simulink library "svm_lib"  (Simulink 8.6)
settings: Solver=VariableStepAuto  StartTime=0.0  StopTime=10.0  RelTol=1e-3
values from neighbouring files (symbols this model uses):
  My_3D = ([eye(6) -eye(6)])    [svm_buildLinearControllers.m]    (also in svm_setup.m = [-eye(6) eye(6)])
  turbulence2loadfactors = blkdiag(T_w2nx, T_w2nz)    [svm_buildLinearControllers.m]
  uavsim = loaded.uavsim    [svm_sandbox.m]
undefined symbols (not defined in the file or in its folder): dt, F, fflib_delay_c2d, Light, mask_p0_NED, mask_v0_NED, MIL, postracking, svm, uavsimblockset_cartesianToAngle
libraries: svm_lib x9, simulink_extras x8, aerolibtransform2 x3, formationFlyingBlockset x2, uavsimBlockset_Cularis_Aerandpropulsion x1, uavsimBlockset_ElectricPropulsion x1, aerolibwind2 x1, aerolibgravity2 x1, uavsimBlockset_VectorNorm x1, uavsimBlockset_UAV3DInterface x1
(part 1 of 3)
settings Model: Creator=j.bolting  LastModifiedBy=j.bolting

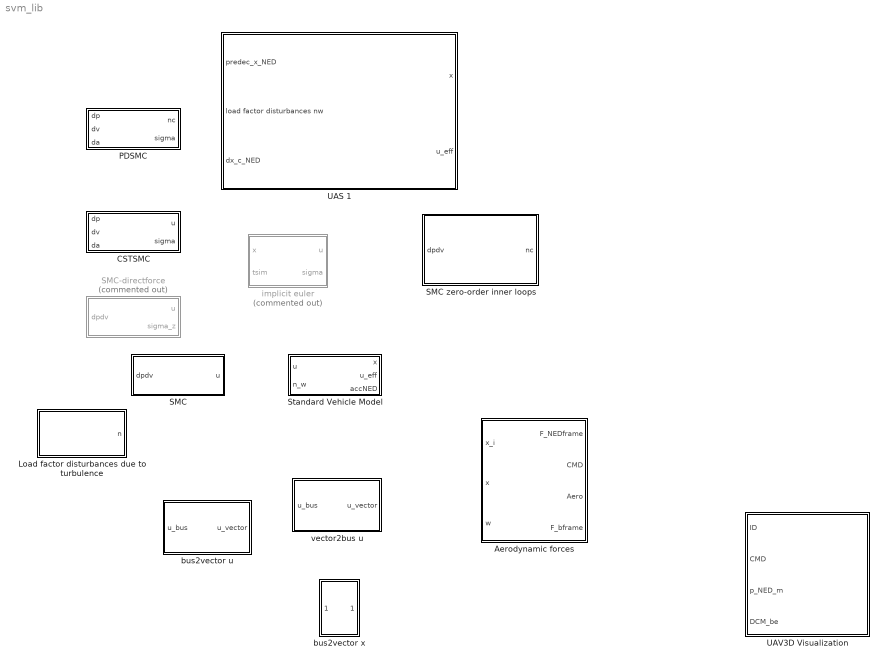
== system svm_lib ==
  Aerodynamic forces : Subsystem
  CSTSMC : Subsystem
  Load factor disturbances due to turbulence : Subsystem
  PDSMC : Subsystem
  SMC : Subsystem
  SMC zero-order inner loops : Subsystem
  SMC-directforce : Subsystem  Commented=on
  Standard Vehicle Model : Subsystem  mask{mask_p0_NED=mask_p0_NED, mask_v0_NED=mask_v0_NED}
      mask prompts: mask_p0_NED "Initial position NED"; mask_v0_NED "Initial velocity NED"
  UAS 1 : Subsystem  mask{mask_vehicleID=1, mask_p0_NED=[0 0 -5], mask_v0_NED=[15 0 0]}
      mask prompts: mask_vehicleID "Vehicle ID"; mask_p0_NED "Initial NED position"; mask_v0_NED "Intial NED speed"
  UAV3D Visualization : Subsystem  AncestorBlock=formationFlyingBlockset/UAV3D Visualization  TreatAsAtomicUnit=on  SystemSampleTime=1/40  mask{mask_visual=2}
      mask prompts: mask_visual "3D model"
      mask TypeOptions mask_visual: 0 | 1 | 2 | 3
  bus2vector u : Subsystem
  bus2vector x : Subsystem
  implicit euler : MATLAB Function  Commented=on  TreatAsAtomicUnit=on  SystemSampleTime=postracking.T
  vector2bus u : Subsystem

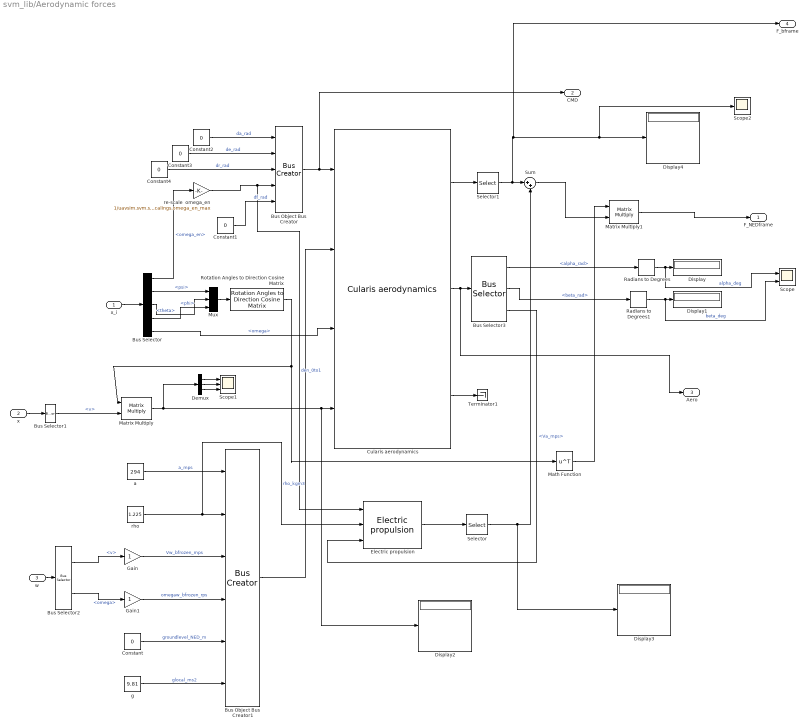
== system svm_lib/Aerodynamic forces ==
  x_i : Inport  OutDataTypeStr=Bus: svm_bus_xi
  x : Inport  Port=2  OutDataTypeStr=Bus: svm_bus_x
  w : Inport  Port=3  OutDataTypeStr=Bus: svm_dwind
  Bus Selector : BusSelector  OutputSignals=omega_en,psi,theta,phi,omega
  Bus Selector1 : BusSelector  OutputSignals=v
  Bus Selector2 : BusSelector  OutputSignals=v,omega
  Bus Selector3 : BusSelector  OutputSignals=alpha_rad,beta_rad,Va_mps
  Bus Object Bus Creator : BusCreator  Inputs=5  OutDataTypeStr=Bus: CMD  mask(BUS OBJECT Bus Creator){busType=Bus: CMD}
      mask prompts: busType "Bus Type"
      mask help:
      | Provides users the cabability to painlessly, instantly customize bus creators of output data type 'Bus:' by selecting the bus object type from a drop down menu dynamically populated by bus objects in the workspace.
      |
      | After pressing the "Apply Selection" button signal lines into the creator are populated and named with the elements in the chosen bus saving the user from having to recall and fill out signal line names.
      |
      | NOTE that when copying a Bus Object Bus Creator from your locked Library the link to the Library is automatically broken. This saves the user from having to Unlock Links To Library (From the Library menu.), Disable Link and finally Break Link (Both from the Model menu.) for every placed instance of the block.
      settings: AttributesFormatString=%<OutDataTypeStr>  CopyFcn=set_param(gcb, 'LinkStatus', 'none')
      mask TypeOptions busType: Bus: AHRS | Bus: Acceleration | Bus: Aero | Bus: Airdata | Bus: Airframe | Bus: Attitude | Bus: CMD | Bus: CMD_quadrotor | Bus: ControlInfoBus | Bus: Enginedata | Bus: Environment | Bus: FlightGearData | Bus: GCSUpstream | Bus: GNSSL1 | Bus: GNSSRTK | Bus: GPS | Bus: IMU | Bus: Kinematics | Bus: LandinggearInput | Bus: MotionTracker | Bus: Position | Bus: Radiodistance | Bus: RotationalAcceleration | Bus: RotationalVelocity | Bus: SensorBus | Bus: StateBus | Bus: Velocity | Bus: WindAngles | Bus: iUAScom | Bus: slBus1 | Bus: svm_bus_u_scaled | Bus: svm_bus_x | Bus: svm_bus_xi | Bus: svm_dwind
      mask Callback busType:
      | % Using variable names terminated with "_BOBC" to lessen the chances of
      | % collisions with existing workspace variables.
      | 
      | % Get the current block handle and mask handle.
      | handleCreator_BOBC = gcbh;
      | maskObj_BOBC       = Simulink.Mask.get(gcb);
      | 
      | % Get a list of variables in the workspace in order to search for the '1x1
      | % Bus' types.
      | wsVars_BOBC = whos;
      | 
      | % Reset the 'TypeOptions' bus list in case some '1x1 Bus' types have been
      | % deleted from or added to the workspace.
      | maskObj_BOBC.Parameters.TypeOptions = {'<empty>'};
      | 
      | % Reset the bus count.
      | busCount_BOBC = 0;
      | 
      | for index_BOBC = 1:length(wsVars_BOBC)
      | 
      |    % If the variable is a bus object...
      |    if strcmp(wsVars_BOBC(index_BOBC).class, 'Simulink.Bus')
      | 
      |       busCount_BOBC = busCount_BOBC + 1;
      | 
      |       % ... add it to the TypeOptions of the mask.
      |       maskObj_BOBC.Parameters.TypeOptions(busCount_BOBC) = ...
      |                                                            ...
      |                                  {['Bus: ', wsVars_BOBC(index_BOBC).name]};
      |    end
      | end
      | 
      | if busCount_BOBC == 0
      | 
      |    % If there are NO bus objects in the workspace then provide a warning
      |    % popup...
      |    warndlg('There are currently no bus objects in the workspace - you have no use for this block. Use a normal Bus Creator instead.')
      | 
      |    % ... and do nothing.
      | elseif ~strcmp(get_param(handleCreator_BOBC, 'OutDataTypeStr'), 'Inherit: auto')
      | 
      |    % If the currently selected bus data type ('OutDataTypeStr') is not
      |    % 'Inherit: auto' (i.e., if we are reopening the mask.) then get the
      |    % current 'OutDataTypeStr' and 'maskVal.' ('maskVal' is the selected
      |    % 'TypeOptions' list member.)
      |    outDatStr_BOBC = get_param(handleCreator_BOBC, 'OutDataTypeStr');
      |    maskVal_BOBC   = get_param(handleCreator_BOBC, 'MaskValues');
      | 
      |    if ~strcmp(outDatStr_BOBC, maskVal_BOBC{1})
      | 
      |       % Upon re-opening the mask if the default 'TypeOptions' list member
      |       % (The first one.) contained in 'maskVal' does not match the
      |       % currently selected bus data type ('OutDataTypeStr') then set the
      |       % 'TypeOptions' list member to the selected bus data type. (Cuts down
      |       % on confusion to have the displayed list member match the selected
      |       % bus data type rather than the first entry.)
      |       set_param(handleCreator_BOBC, 'MaskValues', {outDatStr_BOBC});
      |    end
      | end
      | 
      | % Clean up the workspace.
      | clear  handleCreator_BOBC  maskObj_BOBC     wsVars_BOBC ...
      |             busCount_BOBC    index_BOBC  outDatStr_BOBC ...
      |              maskVal_BOBC
      mask DialogControl applyMOCBSelection Prompt: Apply Selection
      mask DialogControl applyMOCBSelection Callback:
      | % Using variable names terminated with "_BOBC" to lessen the chances of
      | % collisions with existing workspace variables.
      | 
      | % Get the current block, current block handle and mask handle.
      | currentBlock_BOBC  = gcb;
      | handleCreator_BOBC = gcbh;
      | 
      | % Get the desired bus type...
      | desiredBusType_BOBC = get_param(handleCreator_BOBC, 'busType');
      | 
      | % ... and set the 'OutDataTypeStr' to it.
      | set_param(handleCreator_BOBC, 'OutDataTypeStr', desiredBusType_BOBC);
      | 
      | %% First delete any existing lines on the port.
      | % Get the line handles.
      | lh_BOBC = get_param(handleCreator_BOBC, 'LineHandles');
      | 
      | % If any lines exist (Non- -1 line handles.), delete them and start over.
      | if max(lh_BOBC.Inport > 0)
      | 
      |    for index_BOBC = 1:length(lh_BOBC.Inport)
      | 
      |       if lh_BOBC.Inport(index_BOBC) > 0
      | 
      |          delete_line(lh_BOBC.Inport(index_BOBC))
      |       end
      |    end
      | end
      | 
      | %% Then work on adding new lines.
      | 
      | % Get the block path for 'add_line' function.
      | blockPath_BOBC = get_param(handleCreator_BOBC, 'Parent');
      | 
      | % Get the newly selected bus type ('OutDataTypeStr')...
      | mocbBusType_BOBC = get_param(currentBlock_BOBC, 'OutDataTypeStr');
      | 
      | % ... and parse off "Bus: " so the string of the desired bus contained in
      | % 'OutDataTypeStr' matches the raw workspace bus names.
      | mocbBusType_BOBC = mocbBusType_BOBC(6:end);
      | 
      | % Then evaluate the string containing the workspace bus name which will
      | % load the desired bus parameters.
      | busParams_BOBC = eval(mocbBusType_BOBC);
      | 
      | % From the parameters grab the number of lines to add.
      | numLines_BOBC = length(busParams_BOBC.Elements);
      | 
      | % Set the number of inputs of the masked bus creator to the number of lines
      | % to add.
      | set_param(handleCreator_BOBC, 'Inputs', num2str(numLines_BOBC));
      | 
      | % Get (Inputs.) port handles so we can grab the positions of them.
      | ph_BOBC = get_param(handleCreator_BOBC, 'PortHandles');
      | 
      | for index_BOBC = 1:numLines_BOBC
      | 
      |    % Get the position of input port number 'index_BOBC'.
      |    portPos_BOBC = get_param(ph_BOBC.Inport(index_BOBC), 'Position');
      | 
      |    % Add a line from 50 pixels left of the port position to the port
      |    % position. (This must be done because it's the lines that get named,
      |    % not the port positions.)
      |    portLine_BOBC = add_line(blockPath_BOBC, [portPos_BOBC - [50 0]; portPos_BOBC]);
      | 
      |    % Rename the new line to the bus 'index_BOBC-st/nd/rd/th' element name.
      |    set_param(portLine_BOBC, 'Name', busParams_BOBC.Elements(index_BOBC).Name)
      | end
      | 
      | %% Cleanup the workspace.
      | clear    currentBlock_BOBC  handleCreator_BOBC      index_BOBC ...
      |        desiredBusType_BOBC             lh_BOBC  blockPath_BOBC ...
      |           mocbBusType_BOBC      busParams_BOBC   numLines_BOBC ...
      |                    ph_BOBC        portPos_BOBC   portLine_BOBC
  Bus Object Bus Creator1 : BusCreator  Inputs=6  OutDataTypeStr=Bus: Environment  mask(BUS OBJECT Bus Creator){busType=Bus: Environment}
      mask prompts: busType "Bus Type"
      mask help:
      | Provides users the cabability to painlessly, instantly customize bus creators of output data type 'Bus:' by selecting the bus object type from a drop down menu dynamically populated by bus objects in the workspace.
      |
      | After pressing the "Apply Selection" button signal lines into the creator are populated and named with the elements in the chosen bus saving the user from having to recall and fill out signal line names.
      |
      | NOTE that when copying a Bus Object Bus Creator from your locked Library the link to the Library is automatically broken. This saves the user from having to Unlock Links To Library (From the Library menu.), Disable Link and finally Break Link (Both from the Model menu.) for every placed instance of the block.
      settings: AttributesFormatString=%<OutDataTypeStr>  CopyFcn=set_param(gcb, 'LinkStatus', 'none')
      mask TypeOptions busType: Bus: AHRS | Bus: Acceleration | Bus: Aero | Bus: Airdata | Bus: Airframe | Bus: Attitude | Bus: CMD | Bus: CMD_quadrotor | Bus: ControlInfoBus | Bus: Enginedata | Bus: Environment | Bus: FlightGearData | Bus: GCSUpstream | Bus: GNSSL1 | Bus: GNSSRTK | Bus: GPS | Bus: IMU | Bus: Kinematics | Bus: LandinggearInput | Bus: MotionTracker | Bus: Position | Bus: Radiodistance | Bus: RotationalAcceleration | Bus: RotationalVelocity | Bus: SensorBus | Bus: StateBus | Bus: Velocity | Bus: WindAngles | Bus: iUAScom | Bus: slBus1 | Bus: svm_bus_u_scaled | Bus: svm_bus_x | Bus: svm_bus_xi | Bus: svm_dwind
      mask Callback busType:
      | % Using variable names terminated with "_BOBC" to lessen the chances of
      | % collisions with existing workspace variables.
      | 
      | % Get the current block handle and mask handle.
      | handleCreator_BOBC = gcbh;
      | maskObj_BOBC       = Simulink.Mask.get(gcb);
      | 
      | % Get a list of variables in the workspace in order to search for the '1x1
      | % Bus' types.
      | wsVars_BOBC = whos;
      | 
      | % Reset the 'TypeOptions' bus list in case some '1x1 Bus' types have been
      | % deleted from or added to the workspace.
      | maskObj_BOBC.Parameters.TypeOptions = {'<empty>'};
      | 
      | % Reset the bus count.
      | busCount_BOBC = 0;
      | 
      | for index_BOBC = 1:length(wsVars_BOBC)
      | 
      |    % If the variable is a bus object...
      |    if strcmp(wsVars_BOBC(index_BOBC).class, 'Simulink.Bus')
      | 
      |       busCount_BOBC = busCount_BOBC + 1;
      | 
      |       % ... add it to the TypeOptions of the mask.
      |       maskObj_BOBC.Parameters.TypeOptions(busCount_BOBC) = ...
      |                                                            ...
      |                                  {['Bus: ', wsVars_BOBC(index_BOBC).name]};
      |    end
      | end
      | 
      | if busCount_BOBC == 0
      | 
      |    % If there are NO bus objects in the workspace then provide a warning
      |    % popup...
      |    warndlg('There are currently no bus objects in the workspace - you have no use for this block. Use a normal Bus Creator instead.')
      | 
      |    % ... and do nothing.
      | elseif ~strcmp(get_param(handleCreator_BOBC, 'OutDataTypeStr'), 'Inherit: auto')
      | 
      |    % If the currently selected bus data type ('OutDataTypeStr') is not
      |    % 'Inherit: auto' (i.e., if we are reopening the mask.) then get the
      |    % current 'OutDataTypeStr' and 'maskVal.' ('maskVal' is the selected
      |    % 'TypeOptions' list member.)
      |    outDatStr_BOBC = get_param(handleCreator_BOBC, 'OutDataTypeStr');
      |    maskVal_BOBC   = get_param(handleCreator_BOBC, 'MaskValues');
      | 
      |    if ~strcmp(outDatStr_BOBC, maskVal_BOBC{1})
      | 
      |       % Upon re-opening the mask if the default 'TypeOptions' list member
      |       % (The first one.) contained in 'maskVal' does not match the
      |       % currently selected bus data type ('OutDataTypeStr') then set the
      |       % 'TypeOptions' list member to the selected bus data type. (Cuts down
      |       % on confusion to have the displayed list member match the selected
      |       % bus data type rather than the first entry.)
      |       set_param(handleCreator_BOBC, 'MaskValues', {outDatStr_BOBC});
      |    end
      | end
      | 
      | % Clean up the workspace.
      | clear  handleCreator_BOBC  maskObj_BOBC     wsVars_BOBC ...
      |             busCount_BOBC    index_BOBC  outDatStr_BOBC ...
      |              maskVal_BOBC
      mask DialogControl applyMOCBSelection Prompt: Apply Selection
      mask DialogControl applyMOCBSelection Callback:
      | % Using variable names terminated with "_BOBC" to lessen the chances of
      | % collisions with existing workspace variables.
      | 
      | % Get the current block, current block handle and mask handle.
      | currentBlock_BOBC  = gcb;
      | handleCreator_BOBC = gcbh;
      | 
      | % Get the desired bus type...
      | desiredBusType_BOBC = get_param(handleCreator_BOBC, 'busType');
      | 
      | % ... and set the 'OutDataTypeStr' to it.
      | set_param(handleCreator_BOBC, 'OutDataTypeStr', desiredBusType_BOBC);
      | 
      | %% First delete any existing lines on the port.
      | % Get the line handles.
      | lh_BOBC = get_param(handleCreator_BOBC, 'LineHandles');
      | 
      | % If any lines exist (Non- -1 line handles.), delete them and start over.
      | if max(lh_BOBC.Inport > 0)
      | 
      |    for index_BOBC = 1:length(lh_BOBC.Inport)
      | 
      |       if lh_BOBC.Inport(index_BOBC) > 0
      | 
      |          delete_line(lh_BOBC.Inport(index_BOBC))
      |       end
      |    end
      | end
      | 
      | %% Then work on adding new lines.
      | 
      | % Get the block path for 'add_line' function.
      | blockPath_BOBC = get_param(handleCreator_BOBC, 'Parent');
      | 
      | % Get the newly selected bus type ('OutDataTypeStr')...
      | mocbBusType_BOBC = get_param(currentBlock_BOBC, 'OutDataTypeStr');
      | 
      | % ... and parse off "Bus: " so the string of the desired bus contained in
      | % 'OutDataTypeStr' matches the raw workspace bus names.
      | mocbBusType_BOBC = mocbBusType_BOBC(6:end);
      | 
      | % Then evaluate the string containing the workspace bus name which will
      | % load the desired bus parameters.
      | busParams_BOBC = eval(mocbBusType_BOBC);
      | 
      | % From the parameters grab the number of lines to add.
      | numLines_BOBC = length(busParams_BOBC.Elements);
      | 
      | % Set the number of inputs of the masked bus creator to the number of lines
      | % to add.
      | set_param(handleCreator_BOBC, 'Inputs', num2str(numLines_BOBC));
      | 
      | % Get (Inputs.) port handles so we can grab the positions of them.
      | ph_BOBC = get_param(handleCreator_BOBC, 'PortHandles');
      | 
      | for index_BOBC = 1:numLines_BOBC
      | 
      |    % Get the position of input port number 'index_BOBC'.
      |    portPos_BOBC = get_param(ph_BOBC.Inport(index_BOBC), 'Position');
      | 
      |    % Add a line from 50 pixels left of the port position to the port
      |    % position. (This must be done because it's the lines that get named,
      |    % not the port positions.)
      |    portLine_BOBC = add_line(blockPath_BOBC, [portPos_BOBC - [50 0]; portPos_BOBC]);
      | 
      |    % Rename the new line to the bus 'index_BOBC-st/nd/rd/th' element name.
      |    set_param(portLine_BOBC, 'Name', busParams_BOBC.Elements(index_BOBC).Name)
      | end
      | 
      | %% Cleanup the workspace.
      | clear    currentBlock_BOBC  handleCreator_BOBC      index_BOBC ...
      |        desiredBusType_BOBC             lh_BOBC  blockPath_BOBC ...
      |           mocbBusType_BOBC      busParams_BOBC   numLines_BOBC ...
      |                    ph_BOBC        portPos_BOBC   portLine_BOBC
  Constant{,1..4} (5 alike) : Constant  Value=0
  Cularis aerodynamics : uavsimBlockset_Cularis_Aerandpropulsion/Cularis aerodynamics  SystemSampleTime=-1
  Demux : Demux  Outputs=3
  Display{,1..4} (5 alike) : Display
  Electric propulsion : uavsimBlockset_ElectricPropulsion/Electric propulsion  mask_C_prop=uavsim.zagi.engine.C_prop  mask_S_prop=uavsim.zagi.engine.S_prop  mask_k_motor=uavsim.zagi.engine.k_motor
  Gain : Gain
  Gain1 : Gain
  Math Function : Math  Operator=transpose  SaturateOnIntegerOverflow=on
  Matrix Multiply : Product  Multiplication=Matrix(*)
  Matrix Multiply1 : Product  Multiplication=Matrix(*)
  Mux : Mux  Inputs=3
  Radians to Degrees : simulink_extras/Transformations/Radians to Degrees
  Radians to Degrees1 : simulink_extras/Transformations/Radians to Degrees
  Rotation Angles to Direction Cosine Matrix : aerolibtransform2/Rotation Angles to Direction Cosine Matrix  rotationOrder=ZYX
  Scope : Scope  NumInputPorts=2
  Scope1 : Scope  NumInputPorts=3
  Scope2 : Scope
  Selector : Selector  InputPortWidth=6  IndexOptions=Index vector (dialog)  Indices=1:3  OutputSizes=1
  Selector1 : Selector  InputPortWidth=6  IndexOptions=Index vector (dialog)  Indices=1:3  OutputSizes=1
  Sum : Sum  Inputs=|++
  Terminator1 : Terminator
  a : Constant  Value=294
  g : Constant  Value=9.81
  re-scale  omega_en : Gain  Gain=1/uavsim.svm.scalings.omega_en_max
  "rho " : Constant  Value=1.225
  F_NEDframe : Outport
  CMD : Outport  Port=2  OutDataTypeStr=Bus: CMD
  Aero : Outport  Port=3  OutDataTypeStr=Bus: Aero
  F_bframe : Outport  Port=4
  wires:
  Selector1/1 -> Sum/1, Display4/1, Scope2/1, F_bframe/1
  Demux/3 -> Scope1/3
  Demux/1 -> Scope1/1
  Demux/2 -> Scope1/2
  Radians to Degrees1/1 -> Display1/1, Scope/2  "beta_deg"
  Radians to Degrees/1 -> Display/1, Scope/1  "alpha_deg"
  Bus Selector3/2 -> Radians to Degrees1/1  "<beta_rad>"
  Bus Selector3/1 -> Radians to Degrees/1  "<alpha_rad>"
  Bus Selector3/3 -> Electric propulsion/3  "<Va_mps>"
  Bus Selector2/1 -> Gain/1  "<v>"
  Bus Selector2/2 -> Gain1/1  "<omega>"
  Bus Object Bus Creator/1 -> CMD/1, Cularis aerodynamics/1
  Constant2/1 -> Bus Object Bus Creator/1  "da_rad"
  Constant3/1 -> Bus Object Bus Creator/2  "de_rad"
  Constant4/1 -> Bus Object Bus Creator/3  "dr_rad"
  re-scale  omega_en/1 -> Electric propulsion/1, Bus Object Bus Creator/4  "den_0to1"
  Constant1/1 -> Bus Object Bus Creator/5  "df_rad"
  x_i/1 -> Bus Selector/1
  Bus Selector/1 -> re-scale  omega_en/1  "<omega_en>"
  Bus Selector/2 -> Mux/1  "<psi>"
  Cularis aerodynamics/2 -> Aero/1, Bus Selector3/1
  Cularis aerodynamics/3 -> Terminator1/1
  Electric propulsion/1 -> Selector/1
  Matrix Multiply1/1 -> F_NEDframe/1
  Selector/1 -> Sum/2, Display3/1
  Cularis aerodynamics/1 -> Selector1/1
  Bus Selector/5 -> Cularis aerodynamics/3  "<omega>"
  Bus Selector/4 -> Mux/3  "<phi>"
  Bus Selector/3 -> Mux/2  "<theta>"
  Mux/1 -> Rotation Angles to Direction Cosine Matrix/1
  a/1 -> Bus Object Bus Creator1/1  "a_mps"
  "rho "/1 -> Electric propulsion/2, Bus Object Bus Creator1/2  "rho_kgm3"
  Gain/1 -> Bus Object Bus Creator1/3  "Vw_bfrozen_mps"
  Gain1/1 -> Bus Object Bus Creator1/4  "omegaw_bfrozen_rps"
  Constant/1 -> Bus Object Bus Creator1/5  "groundlevel_NED_m"
  g/1 -> Bus Object Bus Creator1/6  "glocal_ms2"
  w/1 -> Bus Selector2/1
  Bus Object Bus Creator1/1 -> Cularis aerodynamics/2
  x/1 -> Bus Selector1/1
  Bus Selector1/1 -> Matrix Multiply/2  "<v>"
  Matrix Multiply/1 -> Cularis aerodynamics/4, Display2/1, Demux/1
  Rotation Angles to Direction Cosine Matrix/1 -> Math Function/1, Matrix Multiply/1
  Math Function/1 -> Matrix Multiply1/1
  Sum/1 -> Matrix Multiply1/2

== system svm_lib/CSTSMC ==
  dp : Inport
  dv : Inport  Port=2
  da : Inport  Port=3
  Integrator : Integrator
  MATLAB Function : MATLAB Function  TreatAsAtomicUnit=on
  Scope : Scope
  Sum : Sum  Inputs=|++
  Zero-Order Hold : ZeroOrderHold  SampleTime=postracking.T
  u : Outport
  sigma : Outport  Port=2
  wires:
  da/1 -> MATLAB Function/3(da)
  Sum/1 -> Zero-Order Hold/1, MATLAB Function/4(u)
  Zero-Order Hold/1 -> u/1
  dv/1 -> MATLAB Function/2(dv)
  MATLAB Function/3(sigma) -> sigma/1
  Integrator/1 -> Sum/2
  MATLAB Function/1(u1) -> Sum/1, Scope/1
  MATLAB Function/2(w) -> Integrator/1
  dp/1 -> MATLAB Function/1(dp)

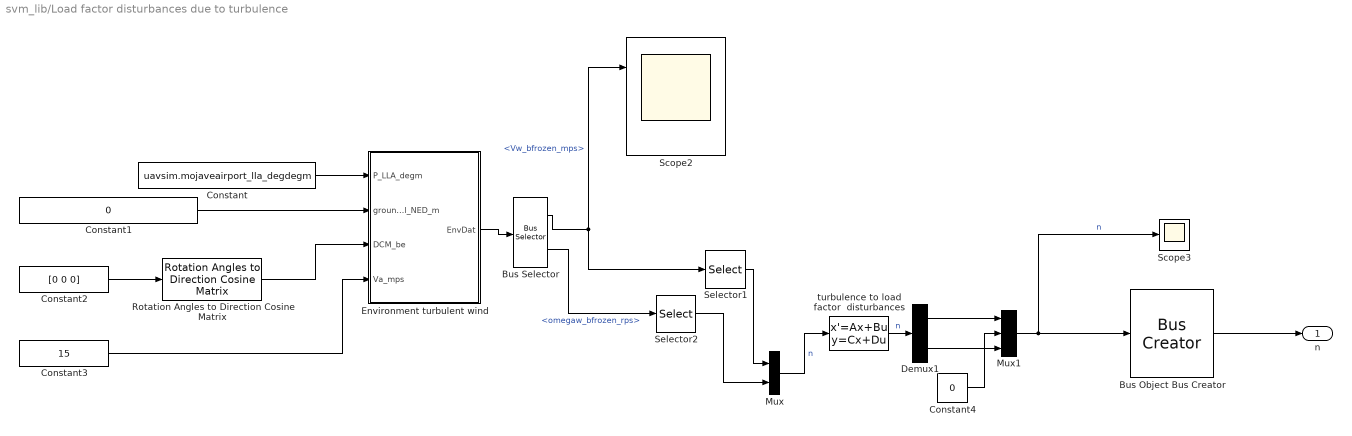
== system svm_lib/Load factor disturbances due to turbulence ==
  Bus Selector : BusSelector  OutputSignals=Vw_bfrozen_mps,omegaw_bfrozen_rps
  Bus Object Bus Creator : BusCreator  Inputs=1  OutDataTypeStr=Bus: svm_bus_u_scaled  mask(BUS OBJECT Bus Creator){busType=Bus: svm_bus_u_scaled}
      mask prompts: busType "Bus Type"
      mask help:
      | Provides users the cabability to painlessly, instantly customize bus creators of output data type 'Bus:' by selecting the bus object type from a drop down menu dynamically populated by bus objects in the workspace.
      |
      | After pressing the "Apply Selection" button signal lines into the creator are populated and named with the elements in the chosen bus saving the user from having to recall and fill out signal line names.
      |
      | NOTE that when copying a Bus Object Bus Creator from your locked Library the link to the Library is automatically broken. This saves the user from having to Unlock Links To Library (From the Library menu.), Disable Link and finally Break Link (Both from the Model menu.) for every placed instance of the block.
      settings: AttributesFormatString=%<OutDataTypeStr>  CopyFcn=set_param(gcb, 'LinkStatus', 'none')
      mask TypeOptions busType: Bus: AHRS | Bus: Acceleration | Bus: Aero | Bus: Airdata | Bus: Airframe | Bus: Attitude | Bus: CMD | Bus: CMD_quadrotor | Bus: ControlInfoBus | Bus: Enginedata | Bus: Environment | Bus: FlightGearData | Bus: GCSUpstream | Bus: GNSSL1 | Bus: GNSSRTK | Bus: GPS | Bus: IMU | Bus: Kinematics | Bus: LandinggearInput | Bus: MotionTracker | Bus: Position | Bus: Radiodistance | Bus: RotationalAcceleration | Bus: RotationalVelocity | Bus: SensorBus | Bus: StateBus | Bus: Velocity | Bus: WindAngles | Bus: iUAScom | Bus: svm_bus_d_exo | Bus: svm_bus_u_scaled | Bus: svm_bus_x | Bus: svm_bus_xi
      mask Callback busType:
      | % Using variable names terminated with "_BOBC" to lessen the chances of
      | % collisions with existing workspace variables.
      | 
      | % Get the current block handle and mask handle.
      | handleCreator_BOBC = gcbh;
      | maskObj_BOBC       = Simulink.Mask.get(gcb);
      | 
      | % Get a list of variables in the workspace in order to search for the '1x1
      | % Bus' types.
      | wsVars_BOBC = whos;
      | 
      | % Reset the 'TypeOptions' bus list in case some '1x1 Bus' types have been
      | % deleted from or added to the workspace.
      | maskObj_BOBC.Parameters.TypeOptions = {'<empty>'};
      | 
      | % Reset the bus count.
      | busCount_BOBC = 0;
      | 
      | for index_BOBC = 1:length(wsVars_BOBC)
      | 
      |    % If the variable is a bus object...
      |    if strcmp(wsVars_BOBC(index_BOBC).class, 'Simulink.Bus')
      | 
      |       busCount_BOBC = busCount_BOBC + 1;
      | 
      |       % ... add it to the TypeOptions of the mask.
      |       maskObj_BOBC.Parameters.TypeOptions(busCount_BOBC) = ...
      |                                                            ...
      |                                  {['Bus: ', wsVars_BOBC(index_BOBC).name]};
      |    end
      | end
      | 
      | if busCount_BOBC == 0
      | 
      |    % If there are NO bus objects in the workspace then provide a warning
      |    % popup...
      |    warndlg('There are currently no bus objects in the workspace - you have no use for this block. Use a normal Bus Creator instead.')
      | 
      |    % ... and do nothing.
      | elseif ~strcmp(get_param(handleCreator_BOBC, 'OutDataTypeStr'), 'Inherit: auto')
      | 
      |    % If the currently selected bus data type ('OutDataTypeStr') is not
      |    % 'Inherit: auto' (i.e., if we are reopening the mask.) then get the
      |    % current 'OutDataTypeStr' and 'maskVal.' ('maskVal' is the selected
      |    % 'TypeOptions' list member.)
      |    outDatStr_BOBC = get_param(handleCreator_BOBC, 'OutDataTypeStr');
      |    maskVal_BOBC   = get_param(handleCreator_BOBC, 'MaskValues');
      | 
      |    if ~strcmp(outDatStr_BOBC, maskVal_BOBC{1})
      | 
      |       % Upon re-opening the mask if the default 'TypeOptions' list member
      |       % (The first one.) contained in 'maskVal' does not match the
      |       % currently selected bus data type ('OutDataTypeStr') then set the
      |       % 'TypeOptions' list member to the selected bus data type. (Cuts down
      |       % on confusion to have the displayed list member match the selected
      |       % bus data type rather than the first entry.)
      |       set_param(handleCreator_BOBC, 'MaskValues', {outDatStr_BOBC});
      |    end
      | end
      | 
      | % Clean up the workspace.
      | clear  handleCreator_BOBC  maskObj_BOBC     wsVars_BOBC ...
      |             busCount_BOBC    index_BOBC  outDatStr_BOBC ...
      |              maskVal_BOBC
      mask DialogControl applyMOCBSelection Prompt: Apply Selection
      mask DialogControl applyMOCBSelection Callback:
      | % Using variable names terminated with "_BOBC" to lessen the chances of
      | % collisions with existing workspace variables.
      | 
      | % Get the current block, current block handle and mask handle.
      | currentBlock_BOBC  = gcb;
      | handleCreator_BOBC = gcbh;
      | 
      | % Get the desired bus type...
      | desiredBusType_BOBC = get_param(handleCreator_BOBC, 'busType');
      | 
      | % ... and set the 'OutDataTypeStr' to it.
      | set_param(handleCreator_BOBC, 'OutDataTypeStr', desiredBusType_BOBC);
      | 
      | %% First delete any existing lines on the port.
      | % Get the line handles.
      | lh_BOBC = get_param(handleCreator_BOBC, 'LineHandles');
      | 
      | % If any lines exist (Non- -1 line handles.), delete them and start over.
      | if max(lh_BOBC.Inport > 0)
      | 
      |    for index_BOBC = 1:length(lh_BOBC.Inport)
      | 
      |       if lh_BOBC.Inport(index_BOBC) > 0
      | 
      |          delete_line(lh_BOBC.Inport(index_BOBC))
      |       end
      |    end
      | end
      | 
      | %% Then work on adding new lines.
      | 
      | % Get the block path for 'add_line' function.
      | blockPath_BOBC = get_param(handleCreator_BOBC, 'Parent');
      | 
      | % Get the newly selected bus type ('OutDataTypeStr')...
      | mocbBusType_BOBC = get_param(currentBlock_BOBC, 'OutDataTypeStr');
      | 
      | % ... and parse off "Bus: " so the string of the desired bus contained in
      | % 'OutDataTypeStr' matches the raw workspace bus names.
      | mocbBusType_BOBC = mocbBusType_BOBC(6:end);
      | 
      | % Then evaluate the string containing the workspace bus name which will
      | % load the desired bus parameters.
      | busParams_BOBC = eval(mocbBusType_BOBC);
      | 
      | % From the parameters grab the number of lines to add.
      | numLines_BOBC = length(busParams_BOBC.Elements);
      | 
      | % Set the number of inputs of the masked bus creator to the number of lines
      | % to add.
      | set_param(handleCreator_BOBC, 'Inputs', num2str(numLines_BOBC));
      | 
      | % Get (Inputs.) port handles so we can grab the positions of them.
      | ph_BOBC = get_param(handleCreator_BOBC, 'PortHandles');
      | 
      | for index_BOBC = 1:numLines_BOBC
      | 
      |    % Get the position of input port number 'index_BOBC'.
      |    portPos_BOBC = get_param(ph_BOBC.Inport(index_BOBC), 'Position');
      | 
      |    % Add a line from 50 pixels left of the port position to the port
      |    % position. (This must be done because it's the lines that get named,
      |    % not the port positions.)
      |    portLine_BOBC = add_line(blockPath_BOBC, [portPos_BOBC - [50 0]; portPos_BOBC]);
      | 
      |    % Rename the new line to the bus 'index_BOBC-st/nd/rd/th' element name.
      |    set_param(portLine_BOBC, 'Name', busParams_BOBC.Elements(index_BOBC).Name)
      | end
      | 
      | %% Cleanup the workspace.
      | clear    currentBlock_BOBC  handleCreator_BOBC      index_BOBC ...
      |        desiredBusType_BOBC             lh_BOBC  blockPath_BOBC ...
      |           mocbBusType_BOBC      busParams_BOBC   numLines_BOBC ...
      |                    ph_BOBC        portPos_BOBC   portLine_BOBC
  Constant : Constant  Value=uavsim.mojaveairport_lla_degdegm
  Constant1 : Constant  Value=0
  Constant2 : Constant  Value=[0 0 0]
  Constant3 : Constant  Value=15
  Constant4 : Constant  Value=0
  Demux1 : Demux  Outputs=2
  Environment turbulent wind : Subsystem  AncestorBlock=uavsimBlockset_Environment_turbulentWind/Environment turbulent wind  mask{mask_constantwind_NED_mps=svm.ambientWind, mask_wingspan=uavsim.cularis.b, mask_windON=svm.ambientWindOn, mask_turbulenceON=svm.turbulenceOn}
      mask prompts: mask_constantwind_NED_mps "Ambient, i.e. constant wind vector [m/s], NED frame"; mask_wingspan "Aircraft wingspan"; mask_windON "Ambient wind ON?"; mask_turbulenceON "Turbulence ON?"
  Mux : Mux  Inputs=2
  Mux1 : Mux  Inputs=3
  Rotation Angles to Direction Cosine Matrix : aerolibtransform2/Rotation Angles to Direction Cosine Matrix  rotationOrder=ZYX
  Scope2 : Scope  NumInputPorts=2
  Scope3 : Scope
  Selector1 : Selector  InputPortWidth=3  IndexOptions=Index vector (dialog)  Indices=[1 3]  OutputSizes=1
  Selector2 : Selector  InputPortWidth=3  IndexOptions=Index vector (dialog)  Indices=2  OutputSizes=1
  turbulence to load factor  disturbances : StateSpace  A=turbulence2loadfactors.a  B=turbulence2loadfactors.b  C=turbulence2loadfactors.c  D=turbulence2loadfactors.d  X0=0
  n : Outport
  wires:
  Selector1/1 -> Mux/1
  Mux/1 -> turbulence to load factor  disturbances/1  "n"
  Bus Object Bus Creator/1 -> n/1
  Constant3/1 -> Environment turbulent wind/4(Va_mps)
  Environment turbulent wind/1(EnvDat) -> Bus Selector/1
  Bus Selector/2 -> Selector2/1  "<omegaw_bfrozen_rps>"
  Rotation Angles to Direction Cosine Matrix/1 -> Environment turbulent wind/3(DCM_be)
  Bus Selector/1 -> Selector1/1, Scope2/1  "<Vw_bfrozen_mps>"
  Constant/1 -> Environment turbulent wind/1(P_LLA_degm)
  Demux1/1 -> Mux1/1
  Constant1/1 -> Environment turbulent wind/2(groundlevel_NED_m)
  turbulence to load factor  disturbances/1 -> Demux1/1  "n"
  Constant2/1 -> Rotation Angles to Direction Cosine Matrix/1
  Selector2/1 -> Mux/2
  Mux1/1 -> Scope3/1, Bus Object Bus Creator/1  "n"
  Demux1/2 -> Mux1/3
  Constant4/1 -> Mux1/2

== system svm_lib/PDSMC ==
  dp : Inport
  dv : Inport  Port=2
  da : Inport  Port=3
  Digital Clock : DigitalClock  SampleTime=-1
  MATLAB Function : MATLAB Function  TreatAsAtomicUnit=on  SystemSampleTime=postracking.T
  Scope : Scope
  Scope1 : Scope
  nc : Outport
  sigma : Outport  Port=2
  wires:
  Digital Clock/1 -> MATLAB Function/4(tsim)
  MATLAB Function/3(dbport) -> Scope1/1
  dp/1 -> MATLAB Function/1(dp)
  MATLAB Function/2(sigma) -> sigma/1
  dv/1 -> MATLAB Function/2(dv)
  MATLAB Function/1(nc) -> Scope/1, nc/1
  da/1 -> MATLAB Function/3(da)

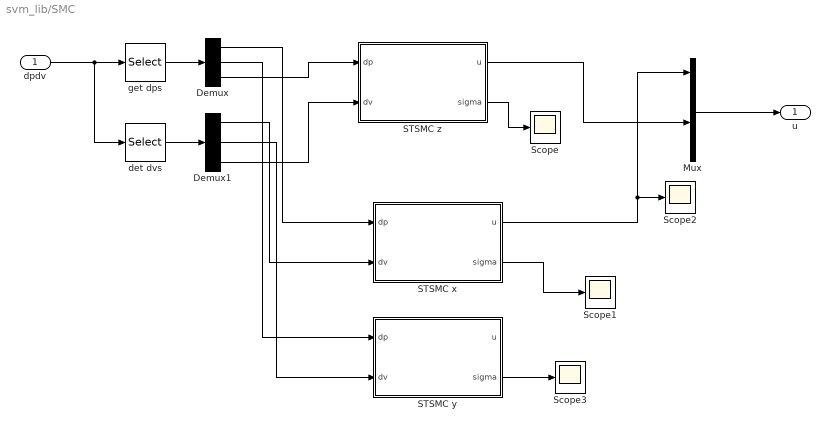
== system svm_lib/SMC ==
  dpdv : Inport
  Demux : Demux  Outputs=3
  Demux1 : Demux  Outputs=3
  Mux : Mux
  STSMC x : Subsystem  SystemSampleTime=postracking.T
  STSMC y : Subsystem  SystemSampleTime=postracking.T
  STSMC z : Subsystem  SystemSampleTime=postracking.T
  Scope{,1..3} (4 alike) : Scope
  det dvs : Selector  InputPortWidth=6  IndexOptions=Index vector (dialog)  Indices=4:6  OutputSizes=1
  get dps : Selector  InputPortWidth=6  IndexOptions=Index vector (dialog)  Indices=1:3  OutputSizes=1
  u : Outport
  wires:
  STSMC y/2(sigma) -> Scope3/1
  ? -> Mux/4
  Demux1/2 -> STSMC y/2(dv)
  Demux/2 -> STSMC y/1(dp)
  STSMC x/2(sigma) -> Scope1/1
  STSMC z/2(sigma) -> Scope/1
  STSMC x/1(u) -> Scope2/1, Mux/1
  Demux1/1 -> STSMC x/2(dv)
  Demux/1 -> STSMC x/1(dp)
  STSMC z/1(u) -> Mux/3
  Mux/1 -> u/1
  Demux1/3 -> STSMC z/2(dv)
  Demux/3 -> STSMC z/1(dp)
  det dvs/1 -> Demux1/1
  get dps/1 -> Demux/1
  dpdv/1 -> get dps/1, det dvs/1

== system svm_lib/SMC zero-order inner loops ==
  dpdv : Inport
  DSMC : Subsystem
  nc : Outport
  wires:
  DSMC/1(nc) -> nc/1
  dpdv/1 -> DSMC/1(dpdv)

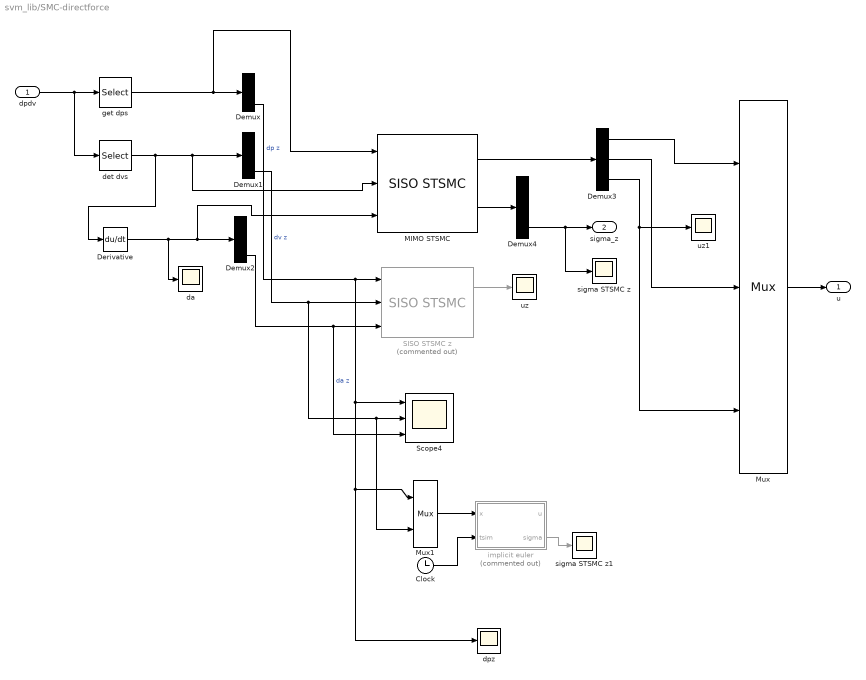
== system svm_lib/SMC-directforce ==
  dpdv : Inport
  Clock : Clock
  Demux{,1..4} (5 alike) : Demux  Outputs=3
  Derivative : Derivative
  MIMO STSMC : svm_lib/SISO STSMC
  Mux : Mux  Inputs=3
  Mux1 : Mux  Inputs=2
  SISO STSMC z : svm_lib/SISO STSMC  Commented=on  mask_k1=-1  mask_k2=-1  mask_lambda=[6; 4; 0]  mask_T=postracking.T  mask_U=1
  Scope4 : Scope  NumInputPorts=3
  da : Scope
  det dvs : Selector  InputPortWidth=6  IndexOptions=Index vector (dialog)  Indices=4:6  OutputSizes=1
  dpz : Scope
  get dps : Selector  InputPortWidth=6  IndexOptions=Index vector (dialog)  Indices=1:3  OutputSizes=1
  implicit euler : MATLAB Function  Commented=on  TreatAsAtomicUnit=on  SystemSampleTime=postracking.T
  sigma STSMC z : Scope
  sigma STSMC z1 : Scope
  uz : Scope
  uz1 : Scope
  u : Outport
  sigma_z : Outport  Port=2
  wires:
  SISO STSMC z/1 -> uz/1
  Demux2/3 -> SISO STSMC z/3, Scope4/3  "da z"
  Derivative/1 -> MIMO STSMC/3, Demux2/1, da/1
  dpdv/1 -> det dvs/1, get dps/1
  get dps/1 -> MIMO STSMC/1, Demux/1
  det dvs/1 -> MIMO STSMC/2, Demux1/1, Derivative/1
  Mux/1 -> u/1
  Demux1/3 -> SISO STSMC z/2, Mux1/2, Scope4/2  "dv z"
  Demux/3 -> SISO STSMC z/1, Mux1/1, dpz/1, Scope4/1  "dp z"
  Mux1/1 -> implicit euler/1(x)
  Clock/1 -> implicit euler/2(tsim)
  implicit euler/2(sigma) -> sigma STSMC z1/1
  MIMO STSMC/1 -> Demux3/1
  Demux3/3 -> Mux/3, uz1/1
  MIMO STSMC/2 -> Demux4/1
  Demux4/3 -> sigma STSMC z/1, sigma_z/1
  Demux3/2 -> Mux/2
  Demux3/1 -> Mux/1

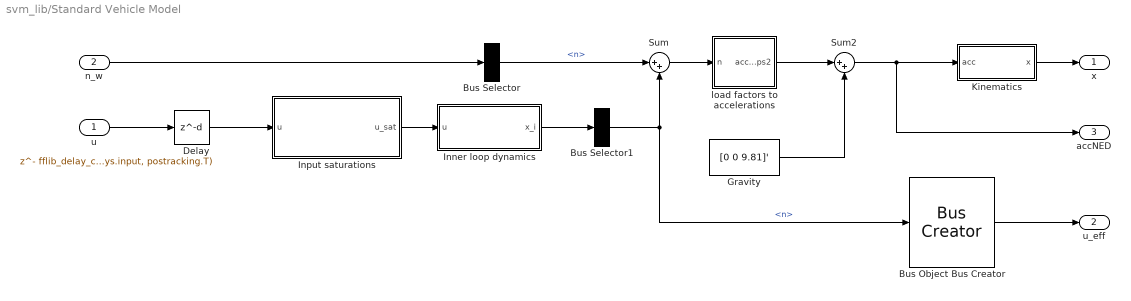
== system svm_lib/Standard Vehicle Model ==
  u : Inport  OutDataTypeStr=Bus: svm_bus_u
  n_w : Inport  Port=2  OutDataTypeStr=Bus: svm_bus_d_exo
  Bus Selector : BusSelector  OutputSignals=n
  Bus Selector1 : BusSelector  OutputSignals=n
  Bus Object Bus Creator : BusCreator  Inputs=1  OutDataTypeStr=Bus: Acceleration  mask(BUS OBJECT Bus Creator){busType=Bus: Acceleration}
      mask prompts: busType "Bus Type"
      mask help:
      | Provides users the cabability to painlessly, instantly customize bus creators of output data type 'Bus:' by selecting the bus object type from a drop down menu dynamically populated by bus objects in the workspace.
      |
      | After pressing the "Apply Selection" button signal lines into the creator are populated and named with the elements in the chosen bus saving the user from having to recall and fill out signal line names.
      |
      | NOTE that when copying a Bus Object Bus Creator from your locked Library the link to the Library is automatically broken. This saves the user from having to Unlock Links To Library (From the Library menu.), Disable Link and finally Break Link (Both from the Model menu.) for every placed instance of the block.
      settings: AttributesFormatString=%<OutDataTypeStr>  CopyFcn=set_param(gcb, 'LinkStatus', 'none')
      mask TypeOptions busType: Bus: Acceleration | Bus: Aero | Bus: Airframe | Bus: Attitude | Bus: CMD | Bus: Environment | Bus: FlightGearData | Bus: Kinematics | Bus: Position | Bus: RotationalAcceleration | Bus: RotationalVelocity | Bus: Velocity | Bus: svm_bus_d_exo | Bus: svm_bus_u | Bus: svm_bus_x | Bus: svm_bus_xi
      mask Callback busType:
      | % Using variable names terminated with "_BOBC" to lessen the chances of
      | % collisions with existing workspace variables.
      | 
      | % Get the current block handle and mask handle.
      | handleCreator_BOBC = gcbh;
      | maskObj_BOBC       = Simulink.Mask.get(gcb);
      | 
      | % Get a list of variables in the workspace in order to search for the '1x1
      | % Bus' types.
      | wsVars_BOBC = whos;
      | 
      | % Reset the 'TypeOptions' bus list in case some '1x1 Bus' types have been
      | % deleted from or added to the workspace.
      | maskObj_BOBC.Parameters.TypeOptions = {'<empty>'};
      | 
      | % Reset the bus count.
      | busCount_BOBC = 0;
      | 
      | for index_BOBC = 1:length(wsVars_BOBC)
      | 
      |    % If the variable is a bus object...
      |    if strcmp(wsVars_BOBC(index_BOBC).class, 'Simulink.Bus')
      | 
      |       busCount_BOBC = busCount_BOBC + 1;
      | 
      |       % ... add it to the TypeOptions of the mask.
      |       maskObj_BOBC.Parameters.TypeOptions(busCount_BOBC) = ...
      |                                                            ...
      |                                  {['Bus: ', wsVars_BOBC(index_BOBC).name]};
      |    end
      | end
      | 
      | if busCount_BOBC == 0
      | 
      |    % If there are NO bus objects in the workspace then provide a warning
      |    % popup...
      |    warndlg('There are currently no bus objects in the workspace - you have no use for this block. Use a normal Bus Creator instead.')
      | 
      |    % ... and do nothing.
      | elseif ~strcmp(get_param(handleCreator_BOBC, 'OutDataTypeStr'), 'Inherit: auto')
      | 
      |    % If the currently selected bus data type ('OutDataTypeStr') is not
      |    % 'Inherit: auto' (i.e., if we are reopening the mask.) then get the
      |    % current 'OutDataTypeStr' and 'maskVal.' ('maskVal' is the selected
      |    % 'TypeOptions' list member.)
      |    outDatStr_BOBC = get_param(handleCreator_BOBC, 'OutDataTypeStr');
      |    maskVal_BOBC   = get_param(handleCreator_BOBC, 'MaskValues');
      | 
      |    if ~strcmp(outDatStr_BOBC, maskVal_BOBC{1})
      | 
      |       % Upon re-opening the mask if the default 'TypeOptions' list member
      |       % (The first one.) contained in 'maskVal' does not match the
      |       % currently selected bus data type ('OutDataTypeStr') then set the
      |       % 'TypeOptions' list member to the selected bus data type. (Cuts down
      |       % on confusion to have the displayed list member match the selected
      |       % bus data type rather than the first entry.)
      |       set_param(handleCreator_BOBC, 'MaskValues', {outDatStr_BOBC});
      |    end
      | end
      | 
      | % Clean up the workspace.
      | clear  handleCreator_BOBC  maskObj_BOBC     wsVars_BOBC ...
      |             busCount_BOBC    index_BOBC  outDatStr_BOBC ...
      |              maskVal_BOBC
      mask DialogControl applyMOCBSelection Prompt: Apply Selection
      mask DialogControl applyMOCBSelection Callback:
      | % Using variable names terminated with "_BOBC" to lessen the chances of
      | % collisions with existing workspace variables.
      | 
      | % Get the current block, current block handle and mask handle.
      | currentBlock_BOBC  = gcb;
      | handleCreator_BOBC = gcbh;
      | 
      | % Get the desired bus type...
      | desiredBusType_BOBC = get_param(handleCreator_BOBC, 'busType');
      | 
      | % ... and set the 'OutDataTypeStr' to it.
      | set_param(handleCreator_BOBC, 'OutDataTypeStr', desiredBusType_BOBC);
      | 
      | %% First delete any existing lines on the port.
      | % Get the line handles.
      | lh_BOBC = get_param(handleCreator_BOBC, 'LineHandles');
      | 
      | % If any lines exist (Non- -1 line handles.), delete them and start over.
      | if max(lh_BOBC.Inport > 0)
      | 
      |    for index_BOBC = 1:length(lh_BOBC.Inport)
      | 
      |       if lh_BOBC.Inport(index_BOBC) > 0
      | 
      |          delete_line(lh_BOBC.Inport(index_BOBC))
      |       end
      |    end
      | end
      | 
      | %% Then work on adding new lines.
      | 
      | % Get the block path for 'add_line' function.
      | blockPath_BOBC = get_param(handleCreator_BOBC, 'Parent');
      | 
      | % Get the newly selected bus type ('OutDataTypeStr')...
      | mocbBusType_BOBC = get_param(currentBlock_BOBC, 'OutDataTypeStr');
      | 
      | % ... and parse off "Bus: " so the string of the desired bus contained in
      | % 'OutDataTypeStr' matches the raw workspace bus names.
      | mocbBusType_BOBC = mocbBusType_BOBC(6:end);
      | 
      | % Then evaluate the string containing the workspace bus name which will
      | % load the desired bus parameters.
      | busParams_BOBC = eval(mocbBusType_BOBC);
      | 
      | % From the parameters grab the number of lines to add.
      | numLines_BOBC = length(busParams_BOBC.Elements);
      | 
      | % Set the number of inputs of the masked bus creator to the number of lines
      | % to add.
      | set_param(handleCreator_BOBC, 'Inputs', num2str(numLines_BOBC));
      | 
      | % Get (Inputs.) port handles so we can grab the positions of them.
      | ph_BOBC = get_param(handleCreator_BOBC, 'PortHandles');
      | 
      | for index_BOBC = 1:numLines_BOBC
      | 
      |    % Get the position of input port number 'index_BOBC'.
      |    portPos_BOBC = get_param(ph_BOBC.Inport(index_BOBC), 'Position');
      | 
      |    % Add a line from 50 pixels left of the port position to the port
      |    % position. (This must be done because it's the lines that get named,
      |    % not the port positions.)
      |    portLine_BOBC = add_line(blockPath_BOBC, [portPos_BOBC - [50 0]; portPos_BOBC]);
      | 
      |    % Rename the new line to the bus 'index_BOBC-st/nd/rd/th' element name.
      |    set_param(portLine_BOBC, 'Name', busParams_BOBC.Elements(index_BOBC).Name)
      | end
      | 
      | %% Cleanup the workspace.
      | clear    currentBlock_BOBC  handleCreator_BOBC      index_BOBC ...
      |        desiredBusType_BOBC             lh_BOBC  blockPath_BOBC ...
      |           mocbBusType_BOBC      busParams_BOBC   numLines_BOBC ...
      |                    ph_BOBC        portPos_BOBC   portLine_BOBC
  Delay : Delay  DelayLength=fflib_delay_c2d(svm.delays.input, postracking.T)
  Gravity : Constant  Value=[0 0 9.81]'
  Inner loop dynamics : Subsystem  Variant=on
  Input saturations : Subsystem
  Kinematics : Subsystem
  Sum : Sum  Inputs=|++
  Sum2 : Sum  Inputs=|++
  load factors to accelerations : Subsystem
  x : Outport  OutDataTypeStr=Bus: svm_bus_x
  u_eff : Outport  Port=2  OutDataTypeStr=Bus: svm_bus_u
  accNED : Outport  Port=3
  wires:
  Bus Selector1/1 -> Bus Object Bus Creator/1, Sum/2  "<n>"
  Delay/1 -> Input saturations/1(u)
  Gravity/1 -> Sum2/2
  Sum2/1 -> Kinematics/1(acc), accNED/1
  load factors to accelerations/1(acc_mps2) -> Sum2/1
  u/1 -> Delay/1
  Kinematics/1(x) -> x/1
  n_w/1 -> Bus Selector/1
  Bus Selector/1 -> Sum/1  "<n>"
  Sum/1 -> load factors to accelerations/1(n)
  Input saturations/1(u_sat) -> Inner loop dynamics/1(u)
  Inner loop dynamics/1(x_i) -> Bus Selector1/1
  Bus Object Bus Creator/1 -> u_eff/1

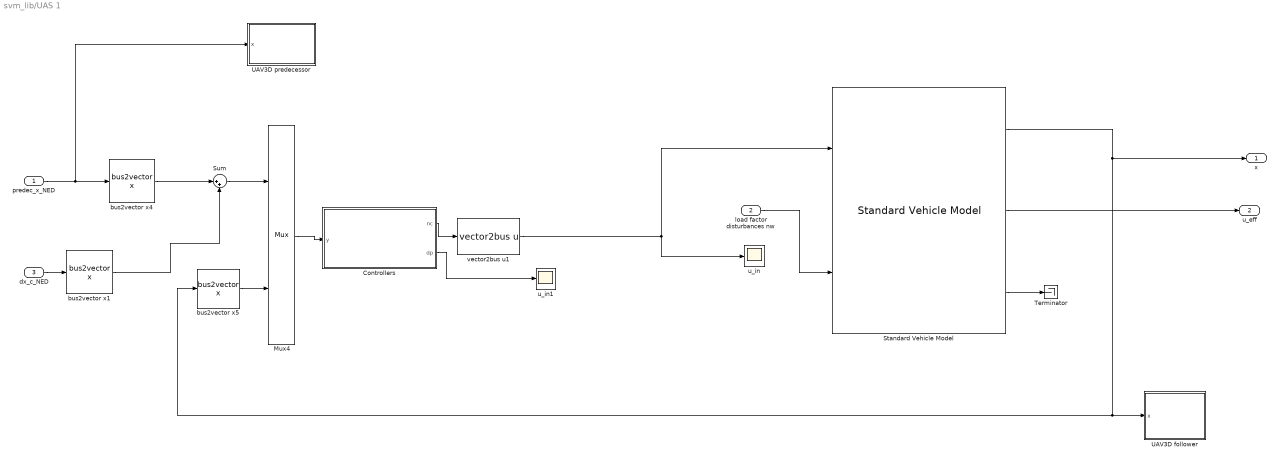
== system svm_lib/UAS 1 ==
  predec_x_NED : Inport  OutDataTypeStr=Bus: svm_bus_x
  load factor disturbances nw : Inport  Port=2  OutDataTypeStr=Bus: svm_bus_u
  dx_c_NED : Inport  Port=3  OutDataTypeStr=Bus: svm_bus_x
  Controllers : Subsystem
  Mux4 : Mux  Inputs=2
  Standard Vehicle Model : svm_lib/Standard Vehicle Model  mask_p0_NED=mask_p0_NED  mask_v0_NED=mask_v0_NED
  Sum : Sum  Inputs=|++
  Terminator : Terminator
  UAV3D follower : Subsystem
  UAV3D predecessor : Subsystem
  bus2vector x1 : svm_lib/bus2vector x
  bus2vector x4 : svm_lib/bus2vector x
  bus2vector x5 : svm_lib/bus2vector x
  u_in : Scope
  u_in1 : Scope
  vector2bus u1 : svm_lib/vector2bus u
  x : Outport  OutDataTypeStr=Bus: svm_bus_x
  u_eff : Outport  Port=2  OutDataTypeStr=Bus: svm_bus_u
  wires:
  Controllers/2(dp) -> u_in1/1
  bus2vector x4/1 -> Sum/1
  Standard Vehicle Model/3 -> Terminator/1
  Standard Vehicle Model/2 -> u_eff/1
  load factor disturbances nw/1 -> Standard Vehicle Model/2
  Mux4/1 -> Controllers/1(y)
  Controllers/1(nc) -> vector2bus u1/1
  predec_x_NED/1 -> UAV3D predecessor/1(x), bus2vector x4/1
  vector2bus u1/1 -> u_in/1, Standard Vehicle Model/1
  bus2vector x5/1 -> Mux4/2
  Standard Vehicle Model/1 -> x/1, UAV3D follower/1(x), bus2vector x5/1
  Sum/1 -> Mux4/1
  dx_c_NED/1 -> bus2vector x1/1
  bus2vector x1/1 -> Sum/2

== system svm_lib/UAV3D Visualization ==
  ID : Inport
  CMD : Inport  Port=2  OutDataTypeStr=Bus: CMD
  p_NED_m : Inport  Port=3
  DCM_be : Inport  Port=4
  Bus Selector2 : BusSelector  OutputSignals=da_rad,de_rad,dr_rad,den_0to1,df_rad
  Demux : Demux  Outputs=3
  Demux1 : Demux
  Direction Cosine Matrix   to  Quaternions : aerolibtransform2/Direction Cosine Matrix  to Quaternions
  ID1 : Constant  Value=mask_visual-1
  UAV3D interface : uavsimBlockset_UAV3DInterface/UAV3D interface  ip='localhost'  udpport=4445
  wires:
  Bus Selector2/5 -> UAV3D interface/13  "<df_rad>"
  Bus Selector2/4 -> UAV3D interface/12  "<den_0to1>"
  Bus Selector2/3 -> UAV3D interface/11  "<dr_rad>"
  Bus Selector2/2 -> UAV3D interface/10  "<de_rad>"
  Bus Selector2/1 -> UAV3D interface/9  "<da_rad>"
  CMD/1 -> Bus Selector2/1
  p_NED_m/1 -> Demux/1
  Demux/3 -> UAV3D interface/4
  Demux/2 -> UAV3D interface/3
  Demux/1 -> UAV3D interface/2
  DCM_be/1 -> Direction Cosine Matrix   to  Quaternions/1
  Demux1/1 -> UAV3D interface/5
  Demux1/2 -> UAV3D interface/6
  Demux1/3 -> UAV3D interface/7
  Demux1/4 -> UAV3D interface/8
  Direction Cosine Matrix   to  Quaternions/1 -> Demux1/1
  ID/1 -> UAV3D interface/1
  ID1/1 -> UAV3D interface/14

== system svm_lib/bus2vector u ==
  u_bus : Inport  OutDataTypeStr=Bus: svm_bus_u_scaled
  Bus Selector : BusSelector  OutputSignals=n
  u_vector : Outport
  wires:
  u_bus/1 -> Bus Selector/1
  Bus Selector/1 -> u_vector/1  "<n>"

== system svm_lib/bus2vector x ==
  x_bus : Inport
  Bus Selector : BusSelector  OutputSignals=p,v
  Mux4 : Mux  Inputs=2
  x_vector : Outport
  wires:
  Bus Selector/1 -> Mux4/1  "<p>"
  Bus Selector/2 -> Mux4/2  "<v>"
  x_bus/1 -> Bus Selector/1
  Mux4/1 -> x_vector/1
